simulink model "model10_oe"  (R2022b)
settings: Solver=VariableStepAuto  StartTime=0.0  StopTime=10000  RelTol=1e-3
libraries: simulink x1
settings Model: Creator=lizey  LastModifiedBy=lizey

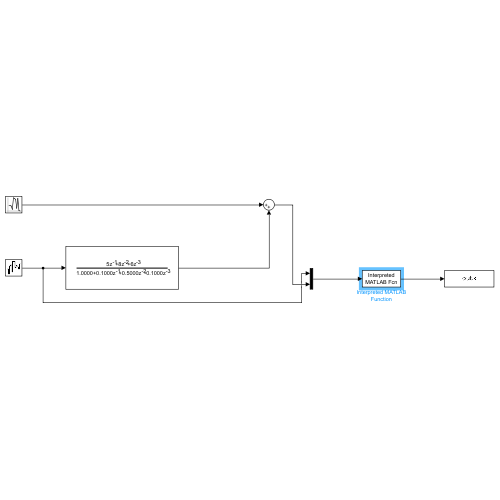
[thumbnail: Simulink's stored preview of the top-level diagram]
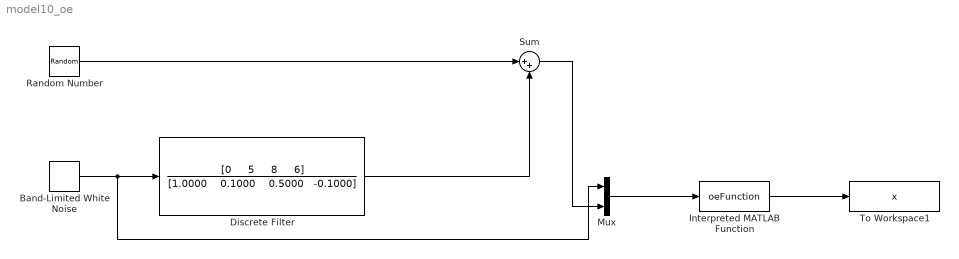
== system model10_oe ==
  Band-Limited White Noise : simulink/Sources/Band-Limited White Noise  Cov=[0.1]  Ts=1  seed=[23341]
  Discrete Filter : DiscreteFilter  Numerator="[0     5     8     6]"  Denominator="[1.0000    0.1000    0.5000   -0.1000]"  SampleTime=1
  Interpreted MATLAB Function : MATLABFcn  MATLABFcn=oeFunction
  Mux : Mux  Inputs=2
  Random Number : RandomNumber  SampleTime=0.1
  Sum : Sum  Inputs=|++
  To Workspace1 : ToWorkspace  VariableName=x  SaveFormat=Timeseries  SampleTime=-1
  wires:
  Band-Limited White Noise/1 -> Mux/1, Discrete Filter/1
  Sum/1 -> Mux/2
  Random Number/1 -> Sum/1
  Discrete Filter/1 -> Sum/2
  Mux/1 -> Interpreted MATLAB Function/1
  Interpreted MATLAB Function/1 -> To Workspace1/1
